simulink model "EZEBsyChk"  (R2018b)
settings: Solver=FixedStepDiscrete  StartTime=0.0  StopTime=10.0  FixedStep=0.01  RelTol=1e-3
settings Model: Creator=sn2xws  LastModifiedBy=sn2xws
settings DataIOCC: SaveFormat=StructureWithTime
settings OptimizationCC: DefaultParameterBehavior=Inlined  EnhancedBackFolding=on  PassReuseOutputArgsAs=Individual arguments  ZeroExternalMemoryAtStartup=off  ZeroInternalMemoryAtStartup=off  OptimizeBlockOrder=speed  DifferentSizesBufferReuse=on  OptimizationCustomize=off
settings DebuggingCC: ParameterTunabilityLossMsg=error
settings ModelReferenceCC: ModelReferenceNumInstancesAllowed=Single
settings SFSimCC: MATLABDynamicMemAlloc=off
settings RTWCC: SystemTargetFile=autosar.tlc  GenCodeOnly=on  TemplateMakefile=ert_default_tmf  Description=AUTOSAR  GenerateReport=on  IncludeHyperlinkInReport=on  LaunchReport=on  GenerateTraceInfo=on  GenerateTraceReport=on  GenerateTraceReportSl=on  GenerateTraceReportSf=on  GenerateTraceReportEml=on
settings CodeAppCC: ForceParamTrailComments=on  IgnoreCustomStorageClasses=off  OperatorAnnotations=on  SimulinkDataObjDesc=on  SFDataObjDesc=on  InsertBlockDesc=on
settings STFCustomTargetCC: TargetLangStandard=C99 (ISO)  MultiwordLength=256  ParMdlRefBuildCompliant=on  CompOptLevelCompliant=on  IncludeMdlTerminateFcn=off  CombineOutputUpdateFcns=on  SuppressErrorStatus=on  ERTCustomFileBanners=on  SupportNonFinite=off  SupportComplex=off  SupportContinuousTime=off  SupportNonInlinedSFcns=off  RemoveResetFunc=on  MATLABClassNameForMDSCustomization=Simulink.SoftwareTarget.ERTCustomization  AutosarCompliant=on  UseToolchainInfoCompliant=on  LookupTableObjectStructAxisOrder=2,1,3,4,...  LUTObjectStructOrderEvenSpacing=Size,Table,Breakpoints  SystemTargetFile=autosar.tlc
settings ERTTargetCC: TargetLangStandard=C99 (ISO)  ConcurrentExecutionCompliant=off  IncludeMdlTerminateFcn=off  SuppressErrorStatus=on  SupportNonFinite=off  SupportComplex=off  ModelStepFunctionPrototypeControlCompliant=off  CPPClassGenCompliant=off  AutosarCompliant=on  LookupTableObjectStructAxisOrder=2,1,3,4,...  LUTObjectStructOrderEvenSpacing=Size,Table,Breakpoints  InlinedParameterPlacement=NonHierarchical  ERTCustomFileTemplate=example_file_process.tlc

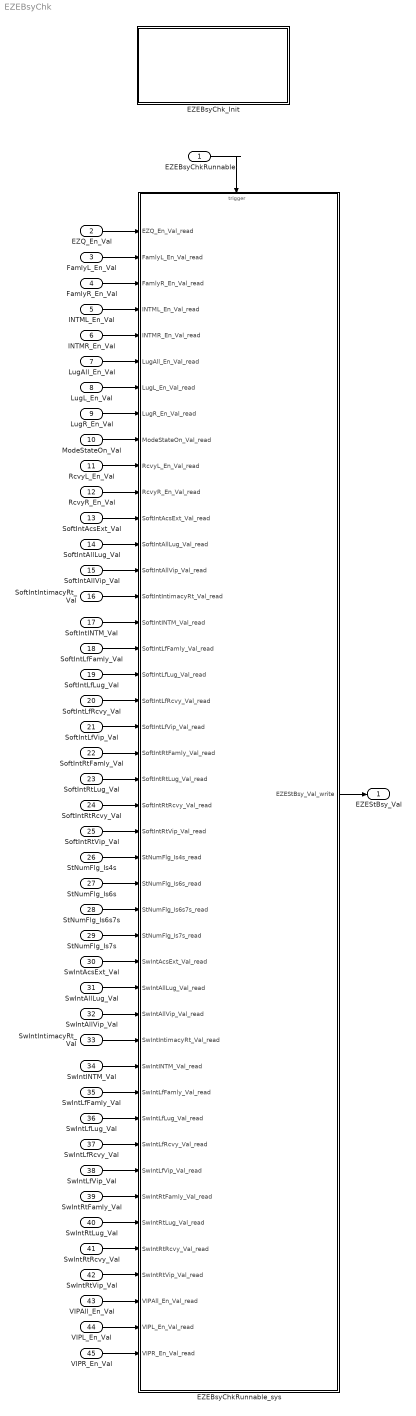
== system EZEBsyChk ==
  EZEBsyChkRunnable : Inport  SampleTime=0.01  OutputFunctionCall=on
  EZQ_En_Val : Inport  Port=2  OutDataTypeStr=boolean  PortDimensions=1
  FamlyL_En_Val : Inport  Port=3  OutDataTypeStr=boolean  PortDimensions=1
  FamlyR_En_Val : Inport  Port=4  OutDataTypeStr=boolean  PortDimensions=1
  INTML_En_Val : Inport  Port=5  OutDataTypeStr=boolean  PortDimensions=1
  INTMR_En_Val : Inport  Port=6  OutDataTypeStr=boolean  PortDimensions=1
  LugAll_En_Val : Inport  Port=7  OutDataTypeStr=boolean  PortDimensions=1
  LugL_En_Val : Inport  Port=8  OutDataTypeStr=boolean  PortDimensions=1
  LugR_En_Val : Inport  Port=9  OutDataTypeStr=boolean  PortDimensions=1
  ModeStateOn_Val : Inport  Port=10  OutDataTypeStr=boolean  PortDimensions=1
  RcvyL_En_Val : Inport  Port=11  OutDataTypeStr=boolean  PortDimensions=1
  RcvyR_En_Val : Inport  Port=12  OutDataTypeStr=boolean  PortDimensions=1
  SoftIntAcsExt_Val : Inport  Port=13  OutDataTypeStr=IntEnable  PortDimensions=1
  SoftIntAllLug_Val : Inport  Port=14  OutDataTypeStr=IntEnable  PortDimensions=1
  SoftIntAllVip_Val : Inport  Port=15  OutDataTypeStr=IntEnable  PortDimensions=1
  SoftIntIntimacyRt_Val : Inport  Port=16  OutDataTypeStr=IntEnable  PortDimensions=1
  SoftIntINTM_Val : Inport  Port=17  OutDataTypeStr=IntEnable  PortDimensions=1
  SoftIntLfFamly_Val : Inport  Port=18  OutDataTypeStr=IntEnable  PortDimensions=1
  SoftIntLfLug_Val : Inport  Port=19  OutDataTypeStr=IntEnable  PortDimensions=1
  SoftIntLfRcvy_Val : Inport  Port=20  OutDataTypeStr=IntEnable  PortDimensions=1
  SoftIntLfVip_Val : Inport  Port=21  OutDataTypeStr=IntEnable  PortDimensions=1
  SoftIntRtFamly_Val : Inport  Port=22  OutDataTypeStr=IntEnable  PortDimensions=1
  SoftIntRtLug_Val : Inport  Port=23  OutDataTypeStr=IntEnable  PortDimensions=1
  SoftIntRtRcvy_Val : Inport  Port=24  OutDataTypeStr=IntEnable  PortDimensions=1
  SoftIntRtVip_Val : Inport  Port=25  OutDataTypeStr=IntEnable  PortDimensions=1
  StNumFlg_Is4s : Inport  Port=26  OutDataTypeStr=boolean  PortDimensions=1
  StNumFlg_Is6s : Inport  Port=27  OutDataTypeStr=boolean  PortDimensions=1
  StNumFlg_Is6s7s : Inport  Port=28  OutDataTypeStr=boolean  PortDimensions=1
  StNumFlg_Is7s : Inport  Port=29  OutDataTypeStr=boolean  PortDimensions=1
  SwIntAcsExt_Val : Inport  Port=30  OutDataTypeStr=IntEnable  PortDimensions=1
  SwIntAllLug_Val : Inport  Port=31  OutDataTypeStr=IntEnable  PortDimensions=1
  SwIntAllVip_Val : Inport  Port=32  OutDataTypeStr=IntEnable  PortDimensions=1
  SwIntIntimacyRt_Val : Inport  Port=33  OutDataTypeStr=IntEnable  PortDimensions=1
  SwIntINTM_Val : Inport  Port=34  OutDataTypeStr=IntEnable  PortDimensions=1
  SwIntLfFamly_Val : Inport  Port=35  OutDataTypeStr=IntEnable  PortDimensions=1
  SwIntLfLug_Val : Inport  Port=36  OutDataTypeStr=IntEnable  PortDimensions=1
  SwIntLfRcvy_Val : Inport  Port=37  OutDataTypeStr=IntEnable  PortDimensions=1
  SwIntLfVip_Val : Inport  Port=38  OutDataTypeStr=IntEnable  PortDimensions=1
  SwIntRtFamly_Val : Inport  Port=39  OutDataTypeStr=IntEnable  PortDimensions=1
  SwIntRtLug_Val : Inport  Port=40  OutDataTypeStr=IntEnable  PortDimensions=1
  SwIntRtRcvy_Val : Inport  Port=41  OutDataTypeStr=IntEnable  PortDimensions=1
  SwIntRtVip_Val : Inport  Port=42  OutDataTypeStr=IntEnable  PortDimensions=1
  VIPAll_En_Val : Inport  Port=43  OutDataTypeStr=boolean  PortDimensions=1
  VIPL_En_Val : Inport  Port=44  OutDataTypeStr=boolean  PortDimensions=1
  VIPR_En_Val : Inport  Port=45  OutDataTypeStr=boolean  PortDimensions=1
  EZEBsyChkRunnable_sys : Subsystem
  EZEBsyChk_Init : Subsystem
  EZEStBsy_Val : Outport  OutDataTypeStr=boolean  PortDimensions=1
  wires:
  EZQ_En_Val/1 -> EZEBsyChkRunnable_sys/1(EZQ_En_Val_read)
  FamlyL_En_Val/1 -> EZEBsyChkRunnable_sys/2(FamlyL_En_Val_read)
  FamlyR_En_Val/1 -> EZEBsyChkRunnable_sys/3(FamlyR_En_Val_read)
  INTML_En_Val/1 -> EZEBsyChkRunnable_sys/4(INTML_En_Val_read)
  INTMR_En_Val/1 -> EZEBsyChkRunnable_sys/5(INTMR_En_Val_read)
  LugAll_En_Val/1 -> EZEBsyChkRunnable_sys/6(LugAll_En_Val_read)
  LugL_En_Val/1 -> EZEBsyChkRunnable_sys/7(LugL_En_Val_read)
  LugR_En_Val/1 -> EZEBsyChkRunnable_sys/8(LugR_En_Val_read)
  ModeStateOn_Val/1 -> EZEBsyChkRunnable_sys/9(ModeStateOn_Val_read)
  RcvyL_En_Val/1 -> EZEBsyChkRunnable_sys/10(RcvyL_En_Val_read)
  RcvyR_En_Val/1 -> EZEBsyChkRunnable_sys/11(RcvyR_En_Val_read)
  SoftIntAcsExt_Val/1 -> EZEBsyChkRunnable_sys/12(SoftIntAcsExt_Val_read)
  SoftIntAllLug_Val/1 -> EZEBsyChkRunnable_sys/13(SoftIntAllLug_Val_read)
  SoftIntAllVip_Val/1 -> EZEBsyChkRunnable_sys/14(SoftIntAllVip_Val_read)
  SoftIntIntimacyRt_Val/1 -> EZEBsyChkRunnable_sys/15(SoftIntIntimacyRt_Val_read)
  SoftIntINTM_Val/1 -> EZEBsyChkRunnable_sys/16(SoftIntINTM_Val_read)
  SoftIntLfFamly_Val/1 -> EZEBsyChkRunnable_sys/17(SoftIntLfFamly_Val_read)
  SoftIntLfLug_Val/1 -> EZEBsyChkRunnable_sys/18(SoftIntLfLug_Val_read)
  SoftIntLfRcvy_Val/1 -> EZEBsyChkRunnable_sys/19(SoftIntLfRcvy_Val_read)
  SoftIntLfVip_Val/1 -> EZEBsyChkRunnable_sys/20(SoftIntLfVip_Val_read)
  SoftIntRtFamly_Val/1 -> EZEBsyChkRunnable_sys/21(SoftIntRtFamly_Val_read)
  SoftIntRtLug_Val/1 -> EZEBsyChkRunnable_sys/22(SoftIntRtLug_Val_read)
  SoftIntRtRcvy_Val/1 -> EZEBsyChkRunnable_sys/23(SoftIntRtRcvy_Val_read)
  SoftIntRtVip_Val/1 -> EZEBsyChkRunnable_sys/24(SoftIntRtVip_Val_read)
  StNumFlg_Is4s/1 -> EZEBsyChkRunnable_sys/25(StNumFlg_Is4s_read)
  StNumFlg_Is6s/1 -> EZEBsyChkRunnable_sys/26(StNumFlg_Is6s_read)
  StNumFlg_Is6s7s/1 -> EZEBsyChkRunnable_sys/27(StNumFlg_Is6s7s_read)
  StNumFlg_Is7s/1 -> EZEBsyChkRunnable_sys/28(StNumFlg_Is7s_read)
  SwIntAcsExt_Val/1 -> EZEBsyChkRunnable_sys/29(SwIntAcsExt_Val_read)
  SwIntAllLug_Val/1 -> EZEBsyChkRunnable_sys/30(SwIntAllLug_Val_read)
  SwIntAllVip_Val/1 -> EZEBsyChkRunnable_sys/31(SwIntAllVip_Val_read)
  SwIntIntimacyRt_Val/1 -> EZEBsyChkRunnable_sys/32(SwIntIntimacyRt_Val_read)
  SwIntINTM_Val/1 -> EZEBsyChkRunnable_sys/33(SwIntINTM_Val_read)
  SwIntLfFamly_Val/1 -> EZEBsyChkRunnable_sys/34(SwIntLfFamly_Val_read)
  SwIntLfLug_Val/1 -> EZEBsyChkRunnable_sys/35(SwIntLfLug_Val_read)
  SwIntLfRcvy_Val/1 -> EZEBsyChkRunnable_sys/36(SwIntLfRcvy_Val_read)
  SwIntLfVip_Val/1 -> EZEBsyChkRunnable_sys/37(SwIntLfVip_Val_read)
  SwIntRtFamly_Val/1 -> EZEBsyChkRunnable_sys/38(SwIntRtFamly_Val_read)
  SwIntRtLug_Val/1 -> EZEBsyChkRunnable_sys/39(SwIntRtLug_Val_read)
  SwIntRtRcvy_Val/1 -> EZEBsyChkRunnable_sys/40(SwIntRtRcvy_Val_read)
  SwIntRtVip_Val/1 -> EZEBsyChkRunnable_sys/41(SwIntRtVip_Val_read)
  VIPAll_En_Val/1 -> EZEBsyChkRunnable_sys/42(VIPAll_En_Val_read)
  VIPL_En_Val/1 -> EZEBsyChkRunnable_sys/43(VIPL_En_Val_read)
  VIPR_En_Val/1 -> EZEBsyChkRunnable_sys/44(VIPR_En_Val_read)
  EZEBsyChkRunnable_sys/1(EZEStBsy_Val_write) -> EZEStBsy_Val/1
  EZEBsyChkRunnable/1 -> EZEBsyChkRunnable_sys/Trigger

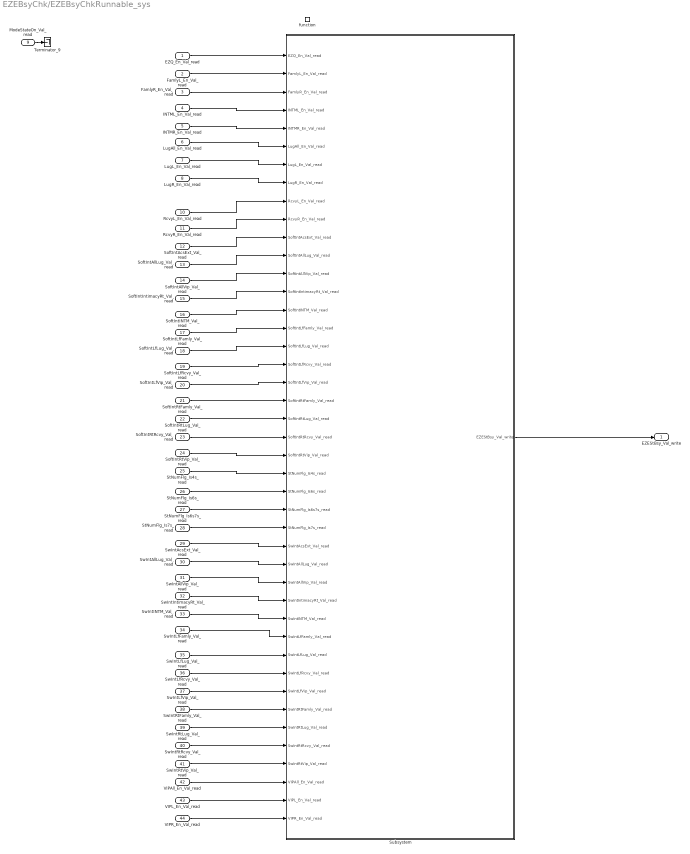
== system EZEBsyChk/EZEBsyChkRunnable_sys ==
  EZQ_En_Val_read : Inport
  FamlyL_En_Val_read : Inport  Port=2
  FamlyR_En_Val_read : Inport  Port=3
  INTML_En_Val_read : Inport  Port=4
  INTMR_En_Val_read : Inport  Port=5
  LugAll_En_Val_read : Inport  Port=6
  LugL_En_Val_read : Inport  Port=7
  LugR_En_Val_read : Inport  Port=8
  ModeStateOn_Val_read : Inport  Port=9
  RcvyL_En_Val_read : Inport  Port=10
  RcvyR_En_Val_read : Inport  Port=11
  SoftIntAcsExt_Val_read : Inport  Port=12
  SoftIntAllLug_Val_read : Inport  Port=13
  SoftIntAllVip_Val_read : Inport  Port=14
  SoftIntIntimacyRt_Val_read : Inport  Port=15
  SoftIntINTM_Val_read : Inport  Port=16
  SoftIntLfFamly_Val_read : Inport  Port=17
  SoftIntLfLug_Val_read : Inport  Port=18
  SoftIntLfRcvy_Val_read : Inport  Port=19
  SoftIntLfVip_Val_read : Inport  Port=20
  SoftIntRtFamly_Val_read : Inport  Port=21
  SoftIntRtLug_Val_read : Inport  Port=22
  SoftIntRtRcvy_Val_read : Inport  Port=23
  SoftIntRtVip_Val_read : Inport  Port=24
  StNumFlg_Is4s_read : Inport  Port=25
  StNumFlg_Is6s_read : Inport  Port=26
  StNumFlg_Is6s7s_read : Inport  Port=27
  StNumFlg_Is7s_read : Inport  Port=28
  SwIntAcsExt_Val_read : Inport  Port=29
  SwIntAllLug_Val_read : Inport  Port=30
  SwIntAllVip_Val_read : Inport  Port=31
  SwIntIntimacyRt_Val_read : Inport  Port=32
  SwIntINTM_Val_read : Inport  Port=33
  SwIntLfFamly_Val_read : Inport  Port=34
  SwIntLfLug_Val_read : Inport  Port=35
  SwIntLfRcvy_Val_read : Inport  Port=36
  SwIntLfVip_Val_read : Inport  Port=37
  SwIntRtFamly_Val_read : Inport  Port=38
  SwIntRtLug_Val_read : Inport  Port=39
  SwIntRtRcvy_Val_read : Inport  Port=40
  SwIntRtVip_Val_read : Inport  Port=41
  VIPAll_En_Val_read : Inport  Port=42
  VIPL_En_Val_read : Inport  Port=43
  VIPR_En_Val_read : Inport  Port=44
  function : TriggerPort  TriggerType=function-call  VariantControl=(inherit)  SampleTimeType=periodic  SampleTime=-1
  Subsystem : Subsystem
  Terminator_9 : Terminator
  EZEStBsy_Val_write : Outport
      settings: EnsureOutportIsVirtual=on
  wires:
  ModeStateOn_Val_read/1 -> Terminator_9/1
  EZQ_En_Val_read/1 -> Subsystem/1(EZQ_En_Val_read)
  FamlyL_En_Val_read/1 -> Subsystem/2(FamlyL_En_Val_read)
  FamlyR_En_Val_read/1 -> Subsystem/3(FamlyR_En_Val_read)
  INTML_En_Val_read/1 -> Subsystem/4(INTML_En_Val_read)
  INTMR_En_Val_read/1 -> Subsystem/5(INTMR_En_Val_read)
  LugAll_En_Val_read/1 -> Subsystem/6(LugAll_En_Val_read)
  LugL_En_Val_read/1 -> Subsystem/7(LugL_En_Val_read)
  LugR_En_Val_read/1 -> Subsystem/8(LugR_En_Val_read)
  RcvyL_En_Val_read/1 -> Subsystem/9(RcvyL_En_Val_read)
  RcvyR_En_Val_read/1 -> Subsystem/10(RcvyR_En_Val_read)
  SoftIntAcsExt_Val_read/1 -> Subsystem/11(SoftIntAcsExt_Val_read)
  SoftIntAllLug_Val_read/1 -> Subsystem/12(SoftIntAllLug_Val_read)
  SoftIntAllVip_Val_read/1 -> Subsystem/13(SoftIntAllVip_Val_read)
  SoftIntIntimacyRt_Val_read/1 -> Subsystem/14(SoftIntIntimacyRt_Val_read)
  SoftIntINTM_Val_read/1 -> Subsystem/15(SoftIntINTM_Val_read)
  SoftIntLfFamly_Val_read/1 -> Subsystem/16(SoftIntLfFamly_Val_read)
  SoftIntLfLug_Val_read/1 -> Subsystem/17(SoftIntLfLug_Val_read)
  SoftIntLfRcvy_Val_read/1 -> Subsystem/18(SoftIntLfRcvy_Val_read)
  SoftIntLfVip_Val_read/1 -> Subsystem/19(SoftIntLfVip_Val_read)
  SoftIntRtFamly_Val_read/1 -> Subsystem/20(SoftIntRtFamly_Val_read)
  SoftIntRtLug_Val_read/1 -> Subsystem/21(SoftIntRtLug_Val_read)
  SoftIntRtRcvy_Val_read/1 -> Subsystem/22(SoftIntRtRcvy_Val_read)
  SoftIntRtVip_Val_read/1 -> Subsystem/23(SoftIntRtVip_Val_read)
  StNumFlg_Is4s_read/1 -> Subsystem/24(StNumFlg_Is4s_read)
  StNumFlg_Is6s_read/1 -> Subsystem/25(StNumFlg_Is6s_read)
  StNumFlg_Is6s7s_read/1 -> Subsystem/26(StNumFlg_Is6s7s_read)
  StNumFlg_Is7s_read/1 -> Subsystem/27(StNumFlg_Is7s_read)
  SwIntAcsExt_Val_read/1 -> Subsystem/28(SwIntAcsExt_Val_read)
  SwIntAllLug_Val_read/1 -> Subsystem/29(SwIntAllLug_Val_read)
  SwIntAllVip_Val_read/1 -> Subsystem/30(SwIntAllVip_Val_read)
  SwIntIntimacyRt_Val_read/1 -> Subsystem/31(SwIntIntimacyRt_Val_read)
  SwIntINTM_Val_read/1 -> Subsystem/32(SwIntINTM_Val_read)
  SwIntLfFamly_Val_read/1 -> Subsystem/33(SwIntLfFamly_Val_read)
  SwIntLfLug_Val_read/1 -> Subsystem/34(SwIntLfLug_Val_read)
  SwIntLfRcvy_Val_read/1 -> Subsystem/35(SwIntLfRcvy_Val_read)
  SwIntLfVip_Val_read/1 -> Subsystem/36(SwIntLfVip_Val_read)
  SwIntRtFamly_Val_read/1 -> Subsystem/37(SwIntRtFamly_Val_read)
  SwIntRtLug_Val_read/1 -> Subsystem/38(SwIntRtLug_Val_read)
  SwIntRtRcvy_Val_read/1 -> Subsystem/39(SwIntRtRcvy_Val_read)
  SwIntRtVip_Val_read/1 -> Subsystem/40(SwIntRtVip_Val_read)
  VIPAll_En_Val_read/1 -> Subsystem/41(VIPAll_En_Val_read)
  VIPL_En_Val_read/1 -> Subsystem/42(VIPL_En_Val_read)
  VIPR_En_Val_read/1 -> Subsystem/43(VIPR_En_Val_read)
  Subsystem/1(EZEStBsy_Val_write) -> EZEStBsy_Val_write/1

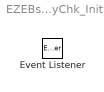
== system EZEBsyChk/EZEBsyChk_Init ==
  Event Listener : EventListener  EventName=reset

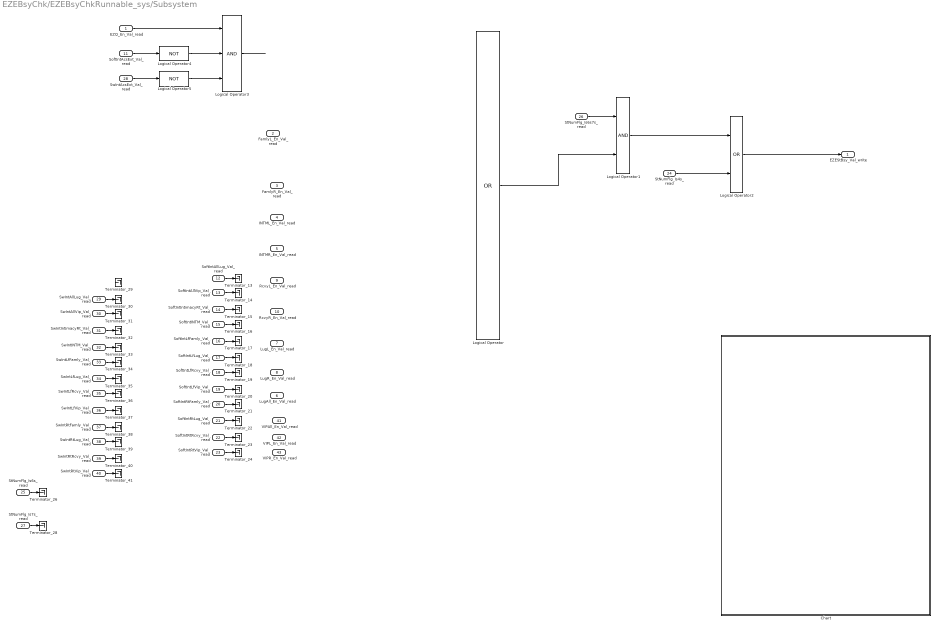
== system EZEBsyChk/EZEBsyChkRunnable_sys/Subsystem ==
  EZQ_En_Val_read : Inport
  FamlyL_En_Val_read : Inport  Port=2
  FamlyR_En_Val_read : Inport  Port=3
  INTML_En_Val_read : Inport  Port=4
  INTMR_En_Val_read : Inport  Port=5
  LugAll_En_Val_read : Inport  Port=6
  LugL_En_Val_read : Inport  Port=7
  LugR_En_Val_read : Inport  Port=8
  RcvyL_En_Val_read : Inport  Port=9
  RcvyR_En_Val_read : Inport  Port=10
  SoftIntAcsExt_Val_read : Inport  Port=11
  SoftIntAllLug_Val_read : Inport  Port=12
  SoftIntAllVip_Val_read : Inport  Port=13
  SoftIntIntimacyRt_Val_read : Inport  Port=14
  SoftIntINTM_Val_read : Inport  Port=15
  SoftIntLfFamly_Val_read : Inport  Port=16
  SoftIntLfLug_Val_read : Inport  Port=17
  SoftIntLfRcvy_Val_read : Inport  Port=18
  SoftIntLfVip_Val_read : Inport  Port=19
  SoftIntRtFamly_Val_read : Inport  Port=20
  SoftIntRtLug_Val_read : Inport  Port=21
  SoftIntRtRcvy_Val_read : Inport  Port=22
  SoftIntRtVip_Val_read : Inport  Port=23
  StNumFlg_Is4s_read : Inport  Port=24
  StNumFlg_Is6s_read : Inport  Port=25
  StNumFlg_Is6s7s_read : Inport  Port=26
  StNumFlg_Is7s_read : Inport  Port=27
  SwIntAcsExt_Val_read : Inport  Port=28
  SwIntAllLug_Val_read : Inport  Port=29
  SwIntAllVip_Val_read : Inport  Port=30
  SwIntIntimacyRt_Val_read : Inport  Port=31
  SwIntINTM_Val_read : Inport  Port=32
  SwIntLfFamly_Val_read : Inport  Port=33
  SwIntLfLug_Val_read : Inport  Port=34
  SwIntLfRcvy_Val_read : Inport  Port=35
  SwIntLfVip_Val_read : Inport  Port=36
  SwIntRtFamly_Val_read : Inport  Port=37
  SwIntRtLug_Val_read : Inport  Port=38
  SwIntRtRcvy_Val_read : Inport  Port=39
  SwIntRtVip_Val_read : Inport  Port=40
  VIPAll_En_Val_read : Inport  Port=41
  VIPL_En_Val_read : Inport  Port=42
  VIPR_En_Val_read : Inport  Port=43
  Chart : Stateflow chart  TreatAsAtomicUnit=on
  Logical Operator : Logic  Operator=OR  Inputs=13  AllPortsSameDT=off  OutDataTypeStr=boolean
  Logical Operator1 : Logic  AllPortsSameDT=off  OutDataTypeStr=boolean
  Logical Operator2 : Logic  Operator=OR  AllPortsSameDT=off  OutDataTypeStr=boolean
  Logical Operator3 : Logic  Inputs=3  AllPortsSameDT=off  OutDataTypeStr=boolean
  Logical Operator4 : Logic  Operator=NOT  Inputs=3  AllPortsSameDT=off  OutDataTypeStr=boolean
  Logical Operator5 : Logic  Operator=NOT  Inputs=3  AllPortsSameDT=off  OutDataTypeStr=boolean
  Terminator_{13..24,26,28..41} (27 alike) : Terminator
  EZEStBsy_Val_write : Outport
      settings: EnsureOutportIsVirtual=on
  wires:
  SwIntLfLug_Val_read/1 -> Terminator_35/1
  StNumFlg_Is6s7s_read/1 -> Logical Operator1/1
  StNumFlg_Is7s_read/1 -> Terminator_28/1
  SoftIntLfLug_Val_read/1 -> Terminator_18/1
  SwIntLfVip_Val_read/1 -> Terminator_37/1
  SoftIntRtFamly_Val_read/1 -> Terminator_21/1
  SwIntRtRcvy_Val_read/1 -> Terminator_40/1
  SwIntAllLug_Val_read/1 -> Terminator_30/1
  SwIntRtFamly_Val_read/1 -> Terminator_38/1
  SwIntRtVip_Val_read/1 -> Terminator_41/1
  SwIntRtLug_Val_read/1 -> Terminator_39/1
  SoftIntLfRcvy_Val_read/1 -> Terminator_19/1
  SoftIntAcsExt_Val_read/1 -> Logical Operator4/1
  SoftIntLfVip_Val_read/1 -> Terminator_20/1
  SoftIntIntimacyRt_Val_read/1 -> Terminator_15/1
  StNumFlg_Is6s_read/1 -> Terminator_26/1
  StNumFlg_Is4s_read/1 -> Logical Operator2/2
  SoftIntINTM_Val_read/1 -> Terminator_16/1
  SoftIntRtRcvy_Val_read/1 -> Terminator_23/1
  SwIntIntimacyRt_Val_read/1 -> Terminator_32/1
  SwIntAllVip_Val_read/1 -> Terminator_31/1
  SwIntINTM_Val_read/1 -> Terminator_33/1
  SwIntLfFamly_Val_read/1 -> Terminator_34/1
  SwIntLfRcvy_Val_read/1 -> Terminator_36/1
  SoftIntLfFamly_Val_read/1 -> Terminator_17/1
  SoftIntAllLug_Val_read/1 -> Terminator_13/1
  SoftIntRtVip_Val_read/1 -> Terminator_24/1
  Logical Operator2/1 -> EZEStBsy_Val_write/1
  SoftIntAllVip_Val_read/1 -> Terminator_14/1
  SoftIntRtLug_Val_read/1 -> Terminator_22/1
  Logical Operator/1 -> Logical Operator1/2
  Logical Operator1/1 -> Logical Operator2/1
  Logical Operator3/1 -> ?
  EZQ_En_Val_read/1 -> Logical Operator3/1
  SwIntAcsExt_Val_read/1 -> Logical Operator5/1
  Logical Operator4/1 -> Logical Operator3/2
  Logical Operator5/1 -> Logical Operator3/3

== stateflow chart EZEBsyChk/EZEBsyChkRunnable_sys/Subsystem/Chart ==
  (default) -> (junction 20)
  (junction 20) -> (junction 17) [order 1] : [is6s||is4s]
  (junction 17) -> (junction 19) [order 1] : [is4s]
  (junction 19) -> ? : {
      | EZEStBsy=1;
      | EZQStBsy=1;
      | LugLStBsy=1;
      | LugRStBsy=1;
      | INTMBsy=1;
      | FamlyLBsy=1;
      | FamlyRBsy=1;
      | INTMRBsy=1;
      | }
  (junction 20) -> (junction 18) [order 2]
  (junction 17) -> (junction 22) [order 2]
  (junction 18) -> (junction 21) [order 1] : [EZQ_En ||VIPL_En||VIPR_En||RecoveryL_En||RecoveryR_En||LugL_En||LugR_En||INTM_En||FAMLY_L_En||FAMLY_R_En||INTMR_En]
  (junction 22) -> (junction 23) [order 1] : [EZQ_En ||VIPL_En||VIPR_En||RecoveryL_En||RecoveryR_En||LugL_En||LugR_En||INTM_En||FAMLY_L_En||FAMLY_R_En||INTMR_En]
  (junction 18) -> (junction 26) [order 2] : {EZEStBsy=0;}
  (junction 21) -> (junction 27) : {EZEStBsy=1;}
  (junction 22) -> (junction 24) [order 2] : {EZEStBsy=0;}
  (junction 23) -> (junction 25) : {EZEStBsy=1;}
  (junction 27) -> (junction 26)
  (junction 25) -> (junction 24)
  (junction 26) -> ?
  (junction 24) -> ?
